simulink model "progetto_simulink"  (R2019b)
settings: Solver=VariableStepAuto  StartTime=0.0  StopTime=1  RelTol=1e-3
values from neighbouring files (symbols this model uses):
  tab_a_inv = 1/tab_a    (= 0.101321183642)    [progetto_3A.m]
  tab_A_n = 0.02    [progetto_3A.m]
  tab_C_d = 2*pi^2    (= 19.7392088022)    [progetto_3A.m]
  tab_eta = 0.6    [progetto_3A.m]
  tab_g_const = 9.80655    [progetto_3A.m]
  tab_omega_n = 1000    [progetto_3A.m]
  tab_R_0 = 45    [progetto_3A.m]
  tab_u_equilibrio = (tab_x_equilibrio_1/(tab_x_equilibrio_2*abs(tab_x_equilibrio_2))-tab_R_0)/(tab_C_d)    [progetto_3A.m]
  tab_W = 30    [progetto_3A.m]
  tab_x_equilibrio_1 = 10    [progetto_3A.m]
  tab_x_equilibrio_2 = 6    [progetto_3A.m]
  tab_x_equilibrio_3 = 6    [progetto_3A.m]
undefined symbols (not defined in the file or in its folder): Den, Num
libraries: cstblocks x2
settings Model: Creator=Luca  LastModifiedBy=Luca

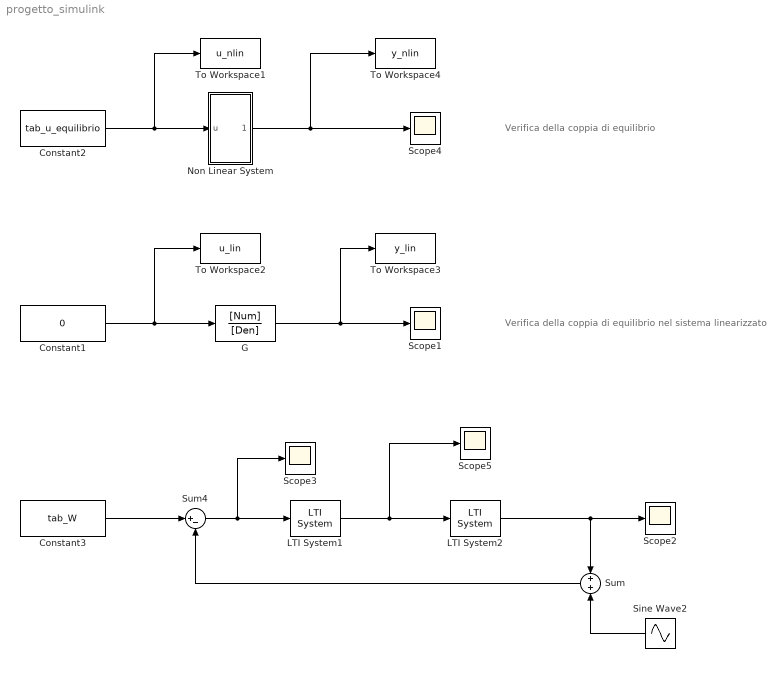
== system progetto_simulink ==
  note: Verifica della coppia di equilibrio
  note: Verifica della coppia di equilibrio nel sistema linearizzato
  Constant1 : Constant  Value=0
  Constant2 : Constant  Value=tab_u_equilibrio
  Constant3 : Constant  Value=tab_W
  G : TransferFcn  Numerator=[Num]  Denominator=[Den]
  LTI System1 : cstblocks/LTI System  sys=R  IC=[]
  LTI System2 : cstblocks/LTI System  sys=G  IC=[]
  Non Linear System : Subsystem
  Scope{1..5} (5 alike) : Scope
  Sine Wave2 : Sin  Amplitude=tab_A_n  Frequency=tab_omega_n  SampleTime=0
  Sum : Sum  Inputs=2
  Sum4 : Sum  Inputs=|+-
  To Workspace1 : ToWorkspace  VariableName=u_nlin  SaveFormat=Timeseries  SampleTime=-1
  To Workspace2 : ToWorkspace  VariableName=u_lin  SaveFormat=Timeseries  SampleTime=-1
  To Workspace3 : ToWorkspace  VariableName=y_lin  SaveFormat=Timeseries  SampleTime=-1
  To Workspace4 : ToWorkspace  VariableName=y_nlin  SaveFormat=Timeseries  SampleTime=-1
  wires:
  Constant2/1 -> Non Linear System/1(u), To Workspace1/1
  G/1 -> To Workspace3/1, Scope1/1
  Constant1/1 -> G/1, To Workspace2/1
  Non Linear System/1(Out1) -> To Workspace4/1, Scope4/1
  LTI System1/1 -> LTI System2/1, Scope5/1
  Sine Wave2/1 -> Sum/2
  LTI System2/1 -> Sum/1, Scope2/1
  Sum/1 -> Sum4/2
  Constant3/1 -> Sum4/1
  Sum4/1 -> Scope3/1, LTI System1/1

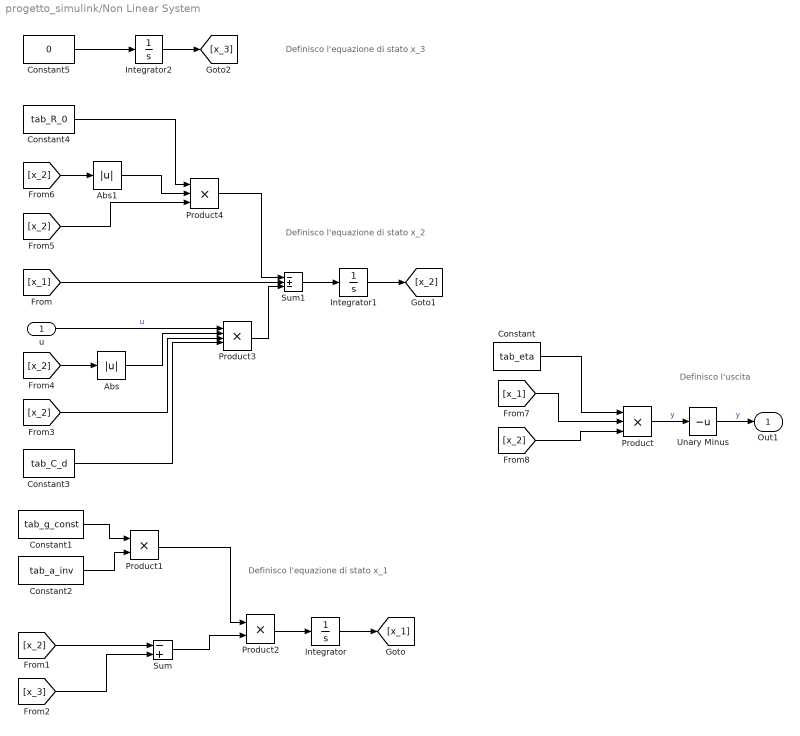
== system progetto_simulink/Non Linear System ==
  note: Definisco l'uscita
  note: Definisco l'equazione di stato x_1
  note: Definisco l'equazione di stato x_3
  note: Definisco l'equazione di stato x_2
  u : Inport
  Abs : Abs
  Abs1 : Abs
  Constant : Constant  Value=tab_eta
  Constant1 : Constant  Value=tab_g_const
  Constant2 : Constant  Value=tab_a_inv
  Constant3 : Constant  Value=tab_C_d
  Constant4 : Constant  Value=tab_R_0
  Constant5 : Constant  Value=0
  Integrator : Integrator  InitialCondition=tab_x_equilibrio_1
  Integrator1 : Integrator  InitialCondition=tab_x_equilibrio_2
  Integrator2 : Integrator  InitialCondition=tab_x_equilibrio_3
  Product : Product  Inputs=3
  Product1 : Product
  Product2 : Product
  Product3 : Product  Inputs=4
  Product4 : Product  Inputs=3
  Sum : Sum  Inputs=-+
  Sum1 : Sum  Inputs=-+-
  Unary Minus : UnaryMinus
  Out1 : Outport
  wires:
  Integrator/1 -> [x_1]
  Integrator1/1 -> [x_2]
  Product1/1 -> Product2/1
  Product3/1 -> Sum1/3
  Product2/1 -> Integrator/1
  [x_2] -> Product/3
  Constant3/1 -> Product3/4
  [x_1] -> Product/2
  Constant5/1 -> Integrator2/1
  Constant1/1 -> Product1/1
  Sum1/1 -> Integrator1/1
  Abs1/1 -> Product4/2
  Constant2/1 -> Product1/2
  Integrator2/1 -> [x_3]
  [x_1] -> Sum1/2
  [x_2] -> Sum/1
  [x_2] -> Abs/1
  Sum/1 -> Product2/2
  Product/1 -> Unary Minus/1  "y"
  Constant4/1 -> Product4/1
  Abs/1 -> Product3/2
  [x_2] -> Product3/3
  u/1 -> Product3/1  "u"
  [x_2] -> Abs1/1
  [x_2] -> Product4/3
  Product4/1 -> Sum1/1
  Constant/1 -> Product/1
  Unary Minus/1 -> Out1/1  "y"
  [x_3] -> Sum/2
